simulink model "waypoint_codegen"  (R2024b)
settings: Solver=FixedStepAuto  StartTime=0.0  StopTime=inf  FixedStep=0.01  RelTol=1e-3
undefined symbols (not defined in the file): X, Y, Z
libraries: robotlib x3, simulink x1, robotcorelib x1, uavalgslib x1
settings Model: SimulationMode=external  Creator=droneproject  LastModifiedBy=droneproject
settings OptimizationCC: DefaultParameterBehavior=Inlined  EnhancedBackFolding=on  PassReuseOutputArgsAs=Individual arguments  ZeroExternalMemoryAtStartup=off  ZeroInternalMemoryAtStartup=off  MaxStackSize=64  OptimizeBlockOrder=speed  DifferentSizesBufferReuse=on  OptimizationCustomize=off  EfficientTunableParamExpr=on
settings DebuggingCC: ParameterTunabilityLossMsg=error
settings HardwareCC: ProdBitPerPointer=32  ProdBitPerSizeT=32  ProdBitPerPtrDiffT=32  ProdLargestAtomicFloat=None  ProdIntDivRoundTo=Undefined  ProdEndianess=Unspecified  ProdWordSize=32  ProdHWDeviceType=Generic->Unspecified (assume 32-bit Generic)  UseEmbeddedCoderFeatures=off
settings SFSimCC: MATLABDynamicMemAlloc=off
settings RTWCC: Description=Embedded Coder  SystemTargetFile=ert.tlc  HardwareBoard=Robot Operating System (ROS)  TLCOptions="-aInlineSetEventsForThisBaseRateFcn=TLC_FALSE -aSuppressMultiTaskScheduler=TLC_FALSE  -aRateBasedStepFcn=0"  GenCodeOnly=on  TemplateMakefile=ert_default_tmf  Toolchain=Catkin  BuildConfiguration=Faster Runs  TargetLang=C++
settings CodeAppCC: ForceParamTrailComments=on  IgnoreCustomStorageClasses=off  OperatorAnnotations=on  SimulinkDataObjDesc=on  SFDataObjDesc=on  InsertBlockDesc=on
settings ERTTargetCC: TargetLangStandard=C++14 (ISO)  SupportNonInlinedSFcns=on

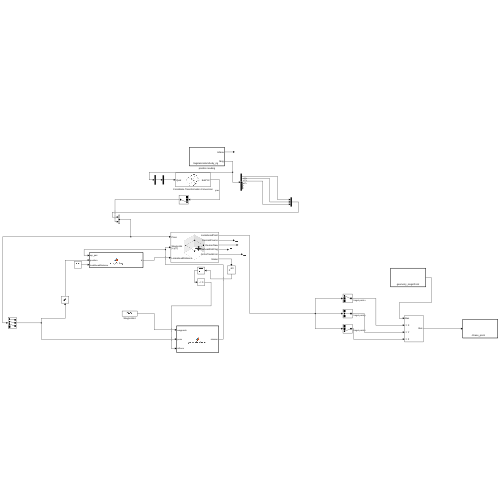
[thumbnail: Simulink's stored preview of the top-level diagram]
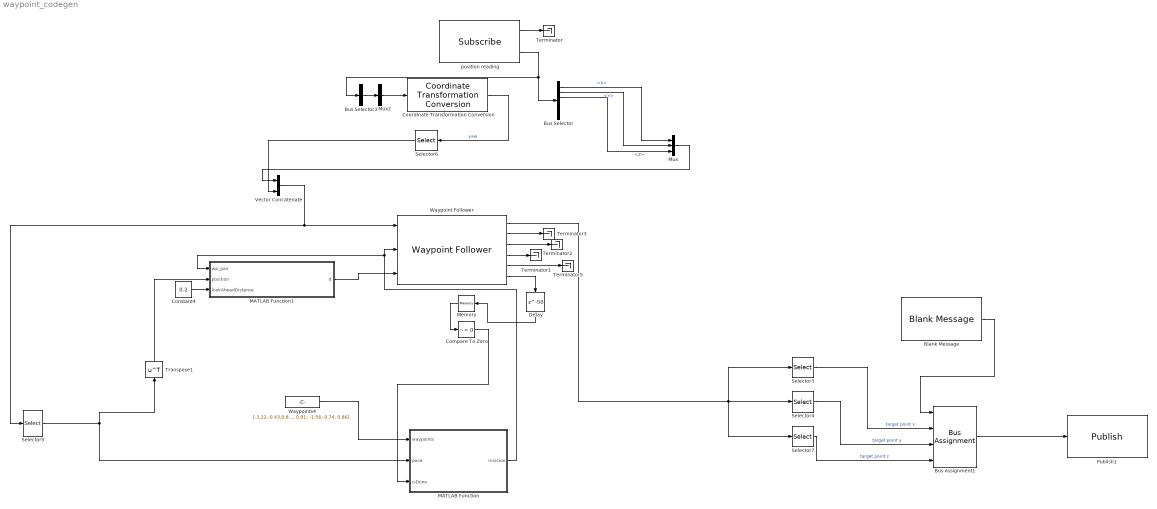
== system waypoint_codegen ==
  Blank Message : robotlib/Blank Message  messageClass=Message  entityType=geometry_msgs/Point  messageType=geometry_msgs/Point  SampleTime=inf  legacyBusStruct=off
  Bus Assignment1 : BusAssignment  AssignedSignals=X,Y,Z
  Bus Selector : BusSelector  DialogController=Simulink.DDGSource_BusSelector  OutputSignals=Pose.Pose.Position.X,Pose.Pose.Position.Y,Pose.Pose.Position.Z,Twist.Twist.Angular.X,Twist.Twist.Angular.Y,Twist.Twist.Angular.Z
  Bus Selector3 : BusSelector  OutputSignals=Pose.Pose.Orientation.X,Pose.Pose.Orientation.Y,Pose.Pose.Orientation.Z,Pose.Pose.Orientation.W  OutputAsBus=on
  Compare To Zero : simulink/Logic and Bit Operations/Compare To Zero  relop=~=  OutDataTypeStr=boolean
  Constant4 : Constant  Value=0.2
  Coordinate Transformation Conversion : robotcorelib/Coordinate Transformation Conversion  InputRepresentation=Quaternion  InputEulerSequence=ZYX  ShowTrVecInputPort=on  OutputRepresentation=Euler Angles  OutputEulerSequence=ZYX  ShowTrVecOutputPort=on  SimulateUsing=Interpreted execution
      settings: LibrarySourceBlock=uavutilslib/Coordinate Transformation Conversion
  Delay : Delay  DelayLength=50  SampleTime=0.01
  MATLAB Function : MATLAB Function  TreatAsAtomicUnit=on
  MATLAB Function1 : MATLAB Function  TreatAsAtomicUnit=on
  Memory : Memory
  Mux : Mux  Inputs=3
  Mux2 : Mux  Inputs=1
  Publish1 : robotlib/Publish  topicSource=Specify your own  topic=/chase_point  messageType=geometry_msgs/Point  legacyBusStruct=off  messageQueueLength=1
  Selector3 : Selector  IndexMode=Zero-based  InputPortWidth=3  IndexOptions=Index vector (dialog)  Indices=[0]  OutputSizes=1
  Selector4 : Selector  IndexMode=Zero-based  InputPortWidth=3  IndexOptions=Index vector (dialog)  Indices=[1]  OutputSizes=1
  Selector5 : Selector  InputPortWidth=4  IndexOptions=Index vector (dialog)  Indices=[1 2 3]  OutputSizes=1
  Selector6 : Selector  InputPortWidth=3  IndexOptions=Index vector (dialog)  Indices=[3]  OutputSizes=1
  Selector7 : Selector  IndexMode=Zero-based  InputPortWidth=3  IndexOptions=Index vector (dialog)  Indices=[2]  OutputSizes=1
  Terminator{,1..3,5} (5 alike) : Terminator
  Transpose1 : Math  Operator=transpose
  Vector Concatenate : Concatenate
  Waypoint Follower : uavalgslib/Waypoint Follower  UAVType=multirotor  StartFrom=first  TransitionRadiusSource=internal  TransitionRadius=0.03  MinLookaheadDistance=0.01  HoverAtLastWaypoint=on  YawInput=off  ShowCrossTrackErrorOutput=on  ShowStatusOutput=on  SimulateUsing=Interpreted execution
  Waypoints4 : Constant  Value=[-3.22,-0.43,0.84; -4.69, -0.40, 1.00; -4.69, 0.54, 1.00; -3.35, 0.51, 0.91; -1.56,-0.74, 0.86]  VectorParams1D=off
  position reading : robotlib/Subscribe  topicSource=Select from ROS network  topic=/tagslam/odom/body_rig  messageType=nav_msgs/Odometry  SampleTime=-1  legacyBusStruct=off  messageQueueLength=1
  wires:
  position reading/2 -> Bus Selector/1, Bus Selector3/1
  position reading/1 -> Terminator/1
  Bus Selector/1 -> Mux/1  "<X>"
  Bus Selector/2 -> Mux/2  "<Y>"
  Bus Selector/3 -> Mux/3  "<Z>"
  Vector Concatenate/1 -> Waypoint Follower/1, Selector5/1
  Waypoint Follower/3 -> Terminator2/1
  Waypoint Follower/2 -> Terminator3/1
  Mux/1 -> Vector Concatenate/1
  MATLAB Function/1(mission) -> Waypoint Follower/2, MATLAB Function1/1(wp_pair)
  Selector5/1 -> Transpose1/1, MATLAB Function/2(pose)
  Transpose1/1 -> MATLAB Function1/2(position)
  Waypoint Follower/5 -> Terminator5/1
  Constant4/1 -> MATLAB Function1/3(lookAheadDistance)
  Waypoint Follower/4 -> Terminator1/1
  Memory/1 -> Compare To Zero/1
  Bus Selector3/1 -> Mux2/1
  Mux2/1 -> Coordinate Transformation Conversion/1
  Coordinate Transformation Conversion/1 -> Selector6/1  "yaw"
  Selector6/1 -> Vector Concatenate/2
  MATLAB Function1/1(d) -> Waypoint Follower/3
  Compare To Zero/1 -> MATLAB Function/3(isDone)
  Waypoint Follower/6 -> Delay/1
  Delay/1 -> Memory/1
  Selector7/1 -> Bus Assignment1/4  "target point z"
  Selector3/1 -> Bus Assignment1/2  "target point x"
  Waypoint Follower/1 -> Selector3/1, Selector7/1, Selector4/1
  Blank Message/1 -> Bus Assignment1/1
  Bus Assignment1/1 -> Publish1/1
  Selector4/1 -> Bus Assignment1/3  "target point y"
  Waypoints4/1 -> MATLAB Function/1(waypoints)

== matlab function waypoint_codegen/MATLAB Function1 ==
  data: wp_pair input; d output; position input; lookAheadDistance input
function d = decayDebug(wp_pair, position, lookAheadDistance)
%#codegen
prevWP = wp_pair(1,:);
nextWP = wp_pair(2,:);

distToStart = norm(position - prevWP);
distToEnd   = norm(position - nextWP);


x = min(distToStart, distToEnd);

if x <= lookAheadDistance
    d = x + 0.02;
else
    d = lookAheadDistance;



end






end

== matlab function waypoint_codegen/MATLAB Function ==
  data: waypoints input; mission output; pose input; isDone input
% MATLAB Function Block: generateMission
% Inputs:
%   waypoints   - Nx3 matrix of [x y z] waypoints
%   pose        - 1x3 current [x y z] position
%   isDone      - scalar (0 or 1), indicates waypoint reached
% Output:
%   mission     - 2x3 matrix: [previous_wp; target_wp]

function mission = generateMission(waypoints, pose, isDone)
%#codegen
% Preallocate output for codegen
mission = zeros(2,3,'like',waypoints);

persistent idx prevWP prevDone nWPs

% Initialize or reset on waypoint count change
if isempty(nWPs)
    nWPs = size(waypoints,1);
end
if isempty(idx) || nWPs ~= size(waypoints,1)
    idx      = 1;
    prevWP   = pose;       % start from initial pose
    prevDone = false;
    nWPs     = size(waypoints,1);
end

% Detect rising edge of isDone
if isDone && ~prevDone

    % Advance previous to current target
    prevWP = waypoints(idx, :);
    % Increment index, cap at end
    idx = min(idx + 1, nWPs);
end
% Store current isDone state
prevDone = isDone;

% Output previous and current target waypoints
mission(1, :) = prevWP;
mission(2, :) = waypoints(idx, :);
end
